simulink model "kiem_chung_dong_hoc"  (R2021a)
settings: Solver=FixedStepAuto  StartTime=0.0  StopTime=5  FixedStep=0.01  RelTol=1e-3
values from neighbouring files (symbols this model uses):
  X = Toado(:,1)    [QuydaoK.m]
  Y = Toado(:,2)    [QuydaoK.m]
  Z = Toado(:,3)    [QuydaoK.m]
undefined symbols (not defined in the file or in its folder): smiData
libraries: sm_lib x36, nesl_utility x13, simulink_extras x12
(part 4 of 4)

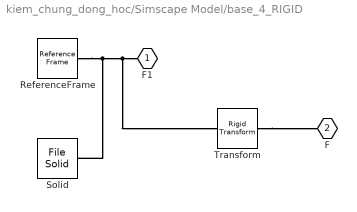
== system kiem_chung_dong_hoc/Simscape Model/base_4_RIGID ==
  ReferenceFrame : sm_lib/Frames and Transforms/Reference Frame
  Solid : sm_lib/Body Elements/File Solid  ExtGeomFileName=base_Default_sldprt.STEP  UnitType=FromFile  ExtGeomFileUnits=m  StepReaderType=HEX  ExportConvexHullGeometry=off  InertiaType=Custom  Mass=smiData.Solid(2).mass  MassUnits=kg  CenterOfMass=smiData.Solid(2).CoM  CenterOfMassUnits=m  MomentsOfInertia=smiData.Solid(2).MoI  MomentsOfInertiaUnits=kg*m^2  ProductsOfInertia=smiData.Solid(2).PoI  ProductsOfInertiaUnits=kg*m^2  BasedOnType=Density  Density=1000  DensityUnits=kg/m^3  DoExposeReferenceFrame=on  SerializedFrames=<Frames/>  GraphicType=FromGeometry  MarkerShape=Sphere  MarkerSize=10  GraphicVisPropType=SimpleVisualProperties  GraphicDiffuseColor=smiData.Solid(2).color  GraphicSpecularColor=[0.5 0.5 0.5 1.0]  GraphicAmbientColor=[0.15 0.15 0.15 1.0]  GraphicEmissiveColor=[0.0 0.0 0.0 1.0]  GraphicShininess=75  GraphicOpacity=smiData.Solid(2).opacity
  Transform : sm_lib/Frames and Transforms/Rigid Transform  TranslationMethod=Cartesian  TranslationStandardOffset=0  TranslationLengthUnit=m  TranslationStandardAxis=+Z  TranslationCartesianOffset=smiData.RigidTransform(3).translation  TranslationROffset=0  TranslationROffsetUnits=m  TranslationZOffset=0  TranslationZOffsetUnits=m  TranslationThetaOffset=0  TranslationThetaOffsetUnits=deg  RotationMethod=ArbitraryAxis  RotationAngleUnits=rad  RotationStandardAxis=+Z  RotationAngle=smiData.RigidTransform(3).angle  RotationArbitraryAxis=smiData.RigidTransform(3).axis  FollAlignAxisA=+X  BaseAlignAxisA=+Y  FollAlignAxisB=+Y  BaseAlignAxisB=+Z  RotationSequenceAxes=FollowerAxes  RotationSequence=XYX  RotationSequenceAngles=[0 0 0]  RotationSequenceAnglesUnits=deg  RotationMatrix=[1 0 0; 0 1 0; 0 0 1]
  F1 : PMIOPort  Side=Left
  F : PMIOPort  Port=2  Side=Right
  connections:
  Solid/RConn1 -- ReferenceFrame/RConn1 -- Transform/LConn1 -- F1/RConn1
  Transform/RConn1 -- F/RConn1

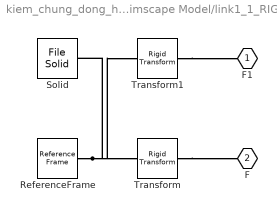
== system kiem_chung_dong_hoc/Simscape Model/link1_1_RIGID ==
  ReferenceFrame : sm_lib/Frames and Transforms/Reference Frame
  Solid : sm_lib/Body Elements/File Solid  ExtGeomFileName=link1_Default_sldprt.STEP  UnitType=FromFile  ExtGeomFileUnits=m  StepReaderType=HEX  ExportConvexHullGeometry=off  InertiaType=Custom  Mass=smiData.Solid(1).mass  MassUnits=kg  CenterOfMass=smiData.Solid(1).CoM  CenterOfMassUnits=m  MomentsOfInertia=smiData.Solid(1).MoI  MomentsOfInertiaUnits=kg*m^2  ProductsOfInertia=smiData.Solid(1).PoI  ProductsOfInertiaUnits=kg*m^2  BasedOnType=Density  Density=1000  DensityUnits=kg/m^3  DoExposeReferenceFrame=on  SerializedFrames=<Frames/>  GraphicType=FromGeometry  MarkerShape=Sphere  MarkerSize=10  GraphicVisPropType=SimpleVisualProperties  GraphicDiffuseColor=smiData.Solid(1).color  GraphicSpecularColor=[0.5 0.5 0.5 1.0]  GraphicAmbientColor=[0.15 0.15 0.15 1.0]  GraphicEmissiveColor=[0.0 0.0 0.0 1.0]  GraphicShininess=75  GraphicOpacity=smiData.Solid(1).opacity
  Transform : sm_lib/Frames and Transforms/Rigid Transform  TranslationMethod=Cartesian  TranslationStandardOffset=0  TranslationLengthUnit=m  TranslationStandardAxis=+Z  TranslationCartesianOffset=smiData.RigidTransform(1).translation  TranslationROffset=0  TranslationROffsetUnits=m  TranslationZOffset=0  TranslationZOffsetUnits=m  TranslationThetaOffset=0  TranslationThetaOffsetUnits=deg  RotationMethod=ArbitraryAxis  RotationAngleUnits=rad  RotationStandardAxis=+Z  RotationAngle=smiData.RigidTransform(1).angle  RotationArbitraryAxis=smiData.RigidTransform(1).axis  FollAlignAxisA=+X  BaseAlignAxisA=+Y  FollAlignAxisB=+Y  BaseAlignAxisB=+Z  RotationSequenceAxes=FollowerAxes  RotationSequence=XYX  RotationSequenceAngles=[0 0 0]  RotationSequenceAnglesUnits=deg  RotationMatrix=[1 0 0; 0 1 0; 0 0 1]
  Transform1 : sm_lib/Frames and Transforms/Rigid Transform  TranslationMethod=Cartesian  TranslationStandardOffset=0  TranslationLengthUnit=m  TranslationStandardAxis=+Z  TranslationCartesianOffset=smiData.RigidTransform(4).translation  TranslationROffset=0  TranslationROffsetUnits=m  TranslationZOffset=0  TranslationZOffsetUnits=m  TranslationThetaOffset=0  TranslationThetaOffsetUnits=deg  RotationMethod=ArbitraryAxis  RotationAngleUnits=rad  RotationStandardAxis=+Z  RotationAngle=smiData.RigidTransform(4).angle  RotationArbitraryAxis=smiData.RigidTransform(4).axis  FollAlignAxisA=+X  BaseAlignAxisA=+Y  FollAlignAxisB=+Y  BaseAlignAxisB=+Z  RotationSequenceAxes=FollowerAxes  RotationSequence=XYX  RotationSequenceAngles=[0 0 0]  RotationSequenceAnglesUnits=deg  RotationMatrix=[1 0 0; 0 1 0; 0 0 1]
  F1 : PMIOPort  Side=Left
  F : PMIOPort  Port=2  Side=Right
  connections:
  Solid/RConn1 -- ReferenceFrame/RConn1 -- Transform/LConn1 -- Transform1/LConn1
  Transform/RConn1 -- F/RConn1
  Transform1/RConn1 -- F1/RConn1

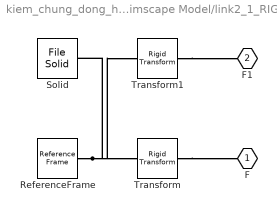
== system kiem_chung_dong_hoc/Simscape Model/link2_1_RIGID ==
  ReferenceFrame : sm_lib/Frames and Transforms/Reference Frame
  Solid : sm_lib/Body Elements/File Solid  ExtGeomFileName=link2_Default_sldprt.STEP  UnitType=FromFile  ExtGeomFileUnits=m  StepReaderType=HEX  ExportConvexHullGeometry=off  InertiaType=Custom  Mass=smiData.Solid(7).mass  MassUnits=kg  CenterOfMass=smiData.Solid(7).CoM  CenterOfMassUnits=m  MomentsOfInertia=smiData.Solid(7).MoI  MomentsOfInertiaUnits=kg*m^2  ProductsOfInertia=smiData.Solid(7).PoI  ProductsOfInertiaUnits=kg*m^2  BasedOnType=Density  Density=1000  DensityUnits=kg/m^3  DoExposeReferenceFrame=on  SerializedFrames=<Frames/>  GraphicType=FromGeometry  MarkerShape=Sphere  MarkerSize=10  GraphicVisPropType=SimpleVisualProperties  GraphicDiffuseColor=smiData.Solid(7).color  GraphicSpecularColor=[0.5 0.5 0.5 1.0]  GraphicAmbientColor=[0.15 0.15 0.15 1.0]  GraphicEmissiveColor=[0.0 0.0 0.0 1.0]  GraphicShininess=75  GraphicOpacity=smiData.Solid(7).opacity
  Transform : sm_lib/Frames and Transforms/Rigid Transform  TranslationMethod=Cartesian  TranslationStandardOffset=0  TranslationLengthUnit=m  TranslationStandardAxis=+Z  TranslationCartesianOffset=smiData.RigidTransform(2).translation  TranslationROffset=0  TranslationROffsetUnits=m  TranslationZOffset=0  TranslationZOffsetUnits=m  TranslationThetaOffset=0  TranslationThetaOffsetUnits=deg  RotationMethod=ArbitraryAxis  RotationAngleUnits=rad  RotationStandardAxis=+Z  RotationAngle=smiData.RigidTransform(2).angle  RotationArbitraryAxis=smiData.RigidTransform(2).axis  FollAlignAxisA=+X  BaseAlignAxisA=+Y  FollAlignAxisB=+Y  BaseAlignAxisB=+Z  RotationSequenceAxes=FollowerAxes  RotationSequence=XYX  RotationSequenceAngles=[0 0 0]  RotationSequenceAnglesUnits=deg  RotationMatrix=[1 0 0; 0 1 0; 0 0 1]
  Transform1 : sm_lib/Frames and Transforms/Rigid Transform  TranslationMethod=Cartesian  TranslationStandardOffset=0  TranslationLengthUnit=m  TranslationStandardAxis=+Z  TranslationCartesianOffset=smiData.RigidTransform(5).translation  TranslationROffset=0  TranslationROffsetUnits=m  TranslationZOffset=0  TranslationZOffsetUnits=m  TranslationThetaOffset=0  TranslationThetaOffsetUnits=deg  RotationMethod=ArbitraryAxis  RotationAngleUnits=rad  RotationStandardAxis=+Z  RotationAngle=smiData.RigidTransform(5).angle  RotationArbitraryAxis=smiData.RigidTransform(5).axis  FollAlignAxisA=+X  BaseAlignAxisA=+Y  FollAlignAxisB=+Y  BaseAlignAxisB=+Z  RotationSequenceAxes=FollowerAxes  RotationSequence=XYX  RotationSequenceAngles=[0 0 0]  RotationSequenceAnglesUnits=deg  RotationMatrix=[1 0 0; 0 1 0; 0 0 1]
  F : PMIOPort  Side=Left
  F1 : PMIOPort  Port=2  Side=Right
  connections:
  Solid/RConn1 -- ReferenceFrame/RConn1 -- Transform/LConn1 -- Transform1/LConn1
  Transform/RConn1 -- F/RConn1
  Transform1/RConn1 -- F1/RConn1

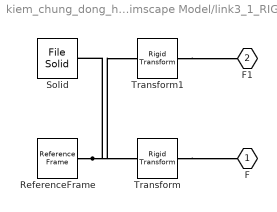
== system kiem_chung_dong_hoc/Simscape Model/link3_1_RIGID ==
  ReferenceFrame : sm_lib/Frames and Transforms/Reference Frame
  Solid : sm_lib/Body Elements/File Solid  ExtGeomFileName=link3_Default_sldprt.STEP  UnitType=FromFile  ExtGeomFileUnits=m  StepReaderType=HEX  ExportConvexHullGeometry=off  InertiaType=Custom  Mass=smiData.Solid(3).mass  MassUnits=kg  CenterOfMass=smiData.Solid(3).CoM  CenterOfMassUnits=m  MomentsOfInertia=smiData.Solid(3).MoI  MomentsOfInertiaUnits=kg*m^2  ProductsOfInertia=smiData.Solid(3).PoI  ProductsOfInertiaUnits=kg*m^2  BasedOnType=Density  Density=1000  DensityUnits=kg/m^3  DoExposeReferenceFrame=on  SerializedFrames=<Frames/>  GraphicType=FromGeometry  MarkerShape=Sphere  MarkerSize=10  GraphicVisPropType=SimpleVisualProperties  GraphicDiffuseColor=smiData.Solid(3).color  GraphicSpecularColor=[0.5 0.5 0.5 1.0]  GraphicAmbientColor=[0.15 0.15 0.15 1.0]  GraphicEmissiveColor=[0.0 0.0 0.0 1.0]  GraphicShininess=75  GraphicOpacity=smiData.Solid(3).opacity
  Transform : sm_lib/Frames and Transforms/Rigid Transform  TranslationMethod=Cartesian  TranslationStandardOffset=0  TranslationLengthUnit=m  TranslationStandardAxis=+Z  TranslationCartesianOffset=smiData.RigidTransform(6).translation  TranslationROffset=0  TranslationROffsetUnits=m  TranslationZOffset=0  TranslationZOffsetUnits=m  TranslationThetaOffset=0  TranslationThetaOffsetUnits=deg  RotationMethod=ArbitraryAxis  RotationAngleUnits=rad  RotationStandardAxis=+Z  RotationAngle=smiData.RigidTransform(6).angle  RotationArbitraryAxis=smiData.RigidTransform(6).axis  FollAlignAxisA=+X  BaseAlignAxisA=+Y  FollAlignAxisB=+Y  BaseAlignAxisB=+Z  RotationSequenceAxes=FollowerAxes  RotationSequence=XYX  RotationSequenceAngles=[0 0 0]  RotationSequenceAnglesUnits=deg  RotationMatrix=[1 0 0; 0 1 0; 0 0 1]
  Transform1 : sm_lib/Frames and Transforms/Rigid Transform  TranslationMethod=Cartesian  TranslationStandardOffset=0  TranslationLengthUnit=m  TranslationStandardAxis=+Z  TranslationCartesianOffset=smiData.RigidTransform(7).translation  TranslationROffset=0  TranslationROffsetUnits=m  TranslationZOffset=0  TranslationZOffsetUnits=m  TranslationThetaOffset=0  TranslationThetaOffsetUnits=deg  RotationMethod=ArbitraryAxis  RotationAngleUnits=rad  RotationStandardAxis=+Z  RotationAngle=smiData.RigidTransform(7).angle  RotationArbitraryAxis=smiData.RigidTransform(7).axis  FollAlignAxisA=+X  BaseAlignAxisA=+Y  FollAlignAxisB=+Y  BaseAlignAxisB=+Z  RotationSequenceAxes=FollowerAxes  RotationSequence=XYX  RotationSequenceAngles=[0 0 0]  RotationSequenceAnglesUnits=deg  RotationMatrix=[1 0 0; 0 1 0; 0 0 1]
  F : PMIOPort  Side=Left
  F1 : PMIOPort  Port=2  Side=Right
  connections:
  Solid/RConn1 -- ReferenceFrame/RConn1 -- Transform/LConn1 -- Transform1/LConn1
  Transform/RConn1 -- F/RConn1
  Transform1/RConn1 -- F1/RConn1

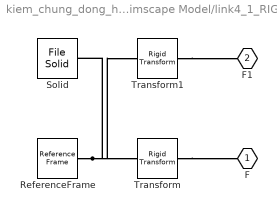
== system kiem_chung_dong_hoc/Simscape Model/link4_1_RIGID ==
  ReferenceFrame : sm_lib/Frames and Transforms/Reference Frame
  Solid : sm_lib/Body Elements/File Solid  ExtGeomFileName=link4_Default_sldprt.STEP  UnitType=FromFile  ExtGeomFileUnits=m  StepReaderType=HEX  ExportConvexHullGeometry=off  InertiaType=Custom  Mass=smiData.Solid(4).mass  MassUnits=kg  CenterOfMass=smiData.Solid(4).CoM  CenterOfMassUnits=m  MomentsOfInertia=smiData.Solid(4).MoI  MomentsOfInertiaUnits=kg*m^2  ProductsOfInertia=smiData.Solid(4).PoI  ProductsOfInertiaUnits=kg*m^2  BasedOnType=Density  Density=1000  DensityUnits=kg/m^3  DoExposeReferenceFrame=on  SerializedFrames=<Frames/>  GraphicType=FromGeometry  MarkerShape=Sphere  MarkerSize=10  GraphicVisPropType=SimpleVisualProperties  GraphicDiffuseColor=smiData.Solid(4).color  GraphicSpecularColor=[0.5 0.5 0.5 1.0]  GraphicAmbientColor=[0.15 0.15 0.15 1.0]  GraphicEmissiveColor=[0.0 0.0 0.0 1.0]  GraphicShininess=75  GraphicOpacity=smiData.Solid(4).opacity
  Transform : sm_lib/Frames and Transforms/Rigid Transform  TranslationMethod=Cartesian  TranslationStandardOffset=0  TranslationLengthUnit=m  TranslationStandardAxis=+Z  TranslationCartesianOffset=smiData.RigidTransform(8).translation  TranslationROffset=0  TranslationROffsetUnits=m  TranslationZOffset=0  TranslationZOffsetUnits=m  TranslationThetaOffset=0  TranslationThetaOffsetUnits=deg  RotationMethod=ArbitraryAxis  RotationAngleUnits=rad  RotationStandardAxis=+Z  RotationAngle=smiData.RigidTransform(8).angle  RotationArbitraryAxis=smiData.RigidTransform(8).axis  FollAlignAxisA=+X  BaseAlignAxisA=+Y  FollAlignAxisB=+Y  BaseAlignAxisB=+Z  RotationSequenceAxes=FollowerAxes  RotationSequence=XYX  RotationSequenceAngles=[0 0 0]  RotationSequenceAnglesUnits=deg  RotationMatrix=[1 0 0; 0 1 0; 0 0 1]
  Transform1 : sm_lib/Frames and Transforms/Rigid Transform  TranslationMethod=Cartesian  TranslationStandardOffset=0  TranslationLengthUnit=m  TranslationStandardAxis=+Z  TranslationCartesianOffset=smiData.RigidTransform(9).translation  TranslationROffset=0  TranslationROffsetUnits=m  TranslationZOffset=0  TranslationZOffsetUnits=m  TranslationThetaOffset=0  TranslationThetaOffsetUnits=deg  RotationMethod=ArbitraryAxis  RotationAngleUnits=rad  RotationStandardAxis=+Z  RotationAngle=smiData.RigidTransform(9).angle  RotationArbitraryAxis=smiData.RigidTransform(9).axis  FollAlignAxisA=+X  BaseAlignAxisA=+Y  FollAlignAxisB=+Y  BaseAlignAxisB=+Z  RotationSequenceAxes=FollowerAxes  RotationSequence=XYX  RotationSequenceAngles=[0 0 0]  RotationSequenceAnglesUnits=deg  RotationMatrix=[1 0 0; 0 1 0; 0 0 1]
  F : PMIOPort  Side=Left
  F1 : PMIOPort  Port=2  Side=Right
  connections:
  Solid/RConn1 -- ReferenceFrame/RConn1 -- Transform/LConn1 -- Transform1/LConn1
  Transform/RConn1 -- F/RConn1
  Transform1/RConn1 -- F1/RConn1

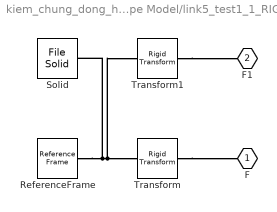
== system kiem_chung_dong_hoc/Simscape Model/link5_test1_1_RIGID ==
  ReferenceFrame : sm_lib/Frames and Transforms/Reference Frame
  Solid : sm_lib/Body Elements/File Solid  ExtGeomFileName=link5_test1_Default_sldprt.STEP  UnitType=FromFile  ExtGeomFileUnits=m  StepReaderType=HEX  ExportConvexHullGeometry=off  InertiaType=Custom  Mass=smiData.Solid(5).mass  MassUnits=kg  CenterOfMass=smiData.Solid(5).CoM  CenterOfMassUnits=m  MomentsOfInertia=smiData.Solid(5).MoI  MomentsOfInertiaUnits=kg*m^2  ProductsOfInertia=smiData.Solid(5).PoI  ProductsOfInertiaUnits=kg*m^2  BasedOnType=Density  Density=1000  DensityUnits=kg/m^3  DoExposeReferenceFrame=on  SerializedFrames=<Frames/>  GraphicType=FromGeometry  MarkerShape=Sphere  MarkerSize=10  GraphicVisPropType=SimpleVisualProperties  GraphicDiffuseColor=smiData.Solid(5).color  GraphicSpecularColor=[0.5 0.5 0.5 1.0]  GraphicAmbientColor=[0.15 0.15 0.15 1.0]  GraphicEmissiveColor=[0.0 0.0 0.0 1.0]  GraphicShininess=75  GraphicOpacity=smiData.Solid(5).opacity
  Transform : sm_lib/Frames and Transforms/Rigid Transform  TranslationMethod=Cartesian  TranslationStandardOffset=0  TranslationLengthUnit=m  TranslationStandardAxis=+Z  TranslationCartesianOffset=smiData.RigidTransform(10).translation  TranslationROffset=0  TranslationROffsetUnits=m  TranslationZOffset=0  TranslationZOffsetUnits=m  TranslationThetaOffset=0  TranslationThetaOffsetUnits=deg  RotationMethod=ArbitraryAxis  RotationAngleUnits=rad  RotationStandardAxis=+Z  RotationAngle=smiData.RigidTransform(10).angle  RotationArbitraryAxis=smiData.RigidTransform(10).axis  FollAlignAxisA=+X  BaseAlignAxisA=+Y  FollAlignAxisB=+Y  BaseAlignAxisB=+Z  RotationSequenceAxes=FollowerAxes  RotationSequence=XYX  RotationSequenceAngles=[0 0 0]  RotationSequenceAnglesUnits=deg  RotationMatrix=[1 0 0; 0 1 0; 0 0 1]
  Transform1 : sm_lib/Frames and Transforms/Rigid Transform  TranslationMethod=Cartesian  TranslationStandardOffset=0  TranslationLengthUnit=m  TranslationStandardAxis=+Z  TranslationCartesianOffset=smiData.RigidTransform(11).translation  TranslationROffset=0  TranslationROffsetUnits=m  TranslationZOffset=0  TranslationZOffsetUnits=m  TranslationThetaOffset=0  TranslationThetaOffsetUnits=deg  RotationMethod=ArbitraryAxis  RotationAngleUnits=rad  RotationStandardAxis=+Z  RotationAngle=smiData.RigidTransform(11).angle  RotationArbitraryAxis=smiData.RigidTransform(11).axis  FollAlignAxisA=+X  BaseAlignAxisA=+Y  FollAlignAxisB=+Y  BaseAlignAxisB=+Z  RotationSequenceAxes=FollowerAxes  RotationSequence=XYX  RotationSequenceAngles=[0 0 0]  RotationSequenceAnglesUnits=deg  RotationMatrix=[1 0 0; 0 1 0; 0 0 1]
  F : PMIOPort  Side=Left
  F1 : PMIOPort  Port=2  Side=Right
  connections:
  Solid/RConn1 -- ReferenceFrame/RConn1 -- Transform/LConn1 -- Transform1/LConn1
  Transform/RConn1 -- F/RConn1
  Transform1/RConn1 -- F1/RConn1

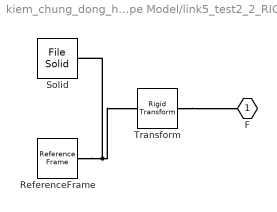
== system kiem_chung_dong_hoc/Simscape Model/link5_test2_2_RIGID ==
  ReferenceFrame : sm_lib/Frames and Transforms/Reference Frame
  Solid : sm_lib/Body Elements/File Solid  ExtGeomFileName=link5_test2_Default_sldprt.STEP  UnitType=FromFile  ExtGeomFileUnits=m  StepReaderType=HEX  ExportConvexHullGeometry=off  InertiaType=Custom  Mass=smiData.Solid(6).mass  MassUnits=kg  CenterOfMass=smiData.Solid(6).CoM  CenterOfMassUnits=m  MomentsOfInertia=smiData.Solid(6).MoI  MomentsOfInertiaUnits=kg*m^2  ProductsOfInertia=smiData.Solid(6).PoI  ProductsOfInertiaUnits=kg*m^2  BasedOnType=Density  Density=1000  DensityUnits=kg/m^3  DoExposeReferenceFrame=on  SerializedFrames=<Frames/>  GraphicType=FromGeometry  MarkerShape=Sphere  MarkerSize=10  GraphicVisPropType=SimpleVisualProperties  GraphicDiffuseColor=smiData.Solid(6).color  GraphicSpecularColor=[0.5 0.5 0.5 1.0]  GraphicAmbientColor=[0.15 0.15 0.15 1.0]  GraphicEmissiveColor=[0.0 0.0 0.0 1.0]  GraphicShininess=75  GraphicOpacity=smiData.Solid(6).opacity
  Transform : sm_lib/Frames and Transforms/Rigid Transform  TranslationMethod=Cartesian  TranslationStandardOffset=0  TranslationLengthUnit=m  TranslationStandardAxis=+Z  TranslationCartesianOffset=smiData.RigidTransform(12).translation  TranslationROffset=0  TranslationROffsetUnits=m  TranslationZOffset=0  TranslationZOffsetUnits=m  TranslationThetaOffset=0  TranslationThetaOffsetUnits=deg  RotationMethod=ArbitraryAxis  RotationAngleUnits=rad  RotationStandardAxis=+Z  RotationAngle=smiData.RigidTransform(12).angle  RotationArbitraryAxis=smiData.RigidTransform(12).axis  FollAlignAxisA=+X  BaseAlignAxisA=+Y  FollAlignAxisB=+Y  BaseAlignAxisB=+Z  RotationSequenceAxes=FollowerAxes  RotationSequence=XYX  RotationSequenceAngles=[0 0 0]  RotationSequenceAnglesUnits=deg  RotationMatrix=[1 0 0; 0 1 0; 0 0 1]
  F : PMIOPort  Side=Left
  connections:
  Solid/RConn1 -- ReferenceFrame/RConn1 -- Transform/LConn1
  Transform/RConn1 -- F/RConn1

== matlab function kiem_chung_dong_hoc/Dong hoc nghich/DONG HOC NGHICH ==
  data: P_EE input; the1 output; the2 output; yaw input; pitch input; roll input; the3 output; the4 output; the5 output; the6 output
% Programmed by Nguyen Ngoc Thien
% Date: 14/07/2022
function [the1,the2,the3,the4,the5,the6] = IK_6DOF(P_EE,yaw,pitch,roll)
%% Thong so cua Robot 6DoF
L2=270; L3=295; L4=80; d1=75; d2=335; d3=90;
% A = [0 0 0 0 0 0;0 0 0 0 0 0;0 0 0 0 0 0;0 0 0 0 0 0;0 0 0 0 0 0;0 0 0 0 0 0;0 0 0 0 0 0;0 0 0 0 0 0];
%% Bo nghiem cua loi giai dong hoc nghich
i = 2;
%% Huong cua Robot
r11 = cosd(yaw)*cosd(pitch);
r12 = cosd(yaw)*sind(pitch)*sind(roll) - sind(yaw)*cosd(roll);
r13 = cosd(yaw)*sind(pitch)*cosd(roll) + sind(yaw)*sind(roll);
r21 = sind(yaw)*cosd(pitch);
r22 = sind(yaw)*sind(pitch)*sind(roll) + cosd(yaw)*cosd(roll);
r23 = sind(yaw)*sind(pitch)*cosd(roll) - cosd(yaw)*sind(roll);
r31 = -sind(pitch);
r32 = cosd(pitch)*sind(roll);
r33 = cosd(pitch)*cosd(roll);
Px = P_EE(1) - L4*r13;
Py = P_EE(2) - L4*r23;
Pz = P_EE(3) - L4*r33;
%% Tinh theta1
s1 = Py/(sqrt(Px^2+Py^2));
c1 = sqrt(1-s1^2);
t1 = [atan2d(s1,c1);
      atan2d(s1,-c1);];
if (i >= 1 && i <= 4)
    the1 = t1(1);
end
if (i >= 5 && i <= 8)
    the1 = t1(2);
end
% for i1 = 1:8
%     A(i1,1) = the1;
% end
%% Tinh theta3
K = ((Px*cosd(the1)+Py*sind(the1)-d1)^2+(Pz-d2)^2-d3^2-L2^2-L3^2)/(2*L2);
t3=[atan2d(d3,L3) - atan2d(K,sqrt(d3^2+L3^2-K^2));
    atan2d(d3,L3) - atan2d(K,-sqrt(d3^2+L3^2-K^2));];
if (i==1 || i==2 || i==5 || i==6)
    the3 = t3(1);
end
if (i==3 || i==4 || i==7 || i==8)
    the3 = t3(2);
end
% for i3 = 1:8
%     A(i3,3) = the3;
% end
%% Tinh theta2
a3=Px*cosd(the1)+Py*sind(the1)-d1;
b3=Pz-d2;
a11=L3*cosd(the3) + d3*sind(the3);
a12=L2 + d3*cosd(the3) - L3*sind(the3);
a21=d3*cosd(the3) - L3*sind(the3) + L2;
a22=-d3*sind(the3) - L3*cosd(the3);
c2=(a3*a22-b3*a12)/(a11*a22-a21*a12);
s2=(a11*b3-a21*a3)/(a11*a22-a21*a12);
the2 = atan2d(s2,c2);
% for i2 = 1:8
%     A(i2,2) = the2;
% end
%% Tinh theta5
c5= r13*cosd(the2 + the3)*cosd(the1) - r33*sind(the2 + the3) + r23*cosd(the2 + the3)*sind(the1);
s5= sqrt(1-c5^2);
t5=[atan2d(s5,c5);
    atan2d(-s5,c5);];
if (i==1 || i==3 || i==5 || i==7)
    the5 = t5(1);
end
if (i==2 || i==4 || i==6 || i==8)
    the5 = t5(2);
end
% for i5 = 1:8
%     A(i5,5) = the5;
% end
%% Tinh theta4
s4=(r23*cosd(the1) - r13*sind(the1))/sind(the5);
c4=-(r33*cosd(the2 + the3) + r13*sind(the2 + the3)*cosd(the1) + r23*sind(the2 + the3)*sind(the1))/sind(the5);
the4 = atan2d(s4,c4);
% for i4 = 1:8
%     A(i4,4) = the4;
% end
%% Tinh theta6
s6= -(r12*cosd(the2 + the3)*cosd(the1) - r32*sind(the2 + the3) + r22*cosd(the2 + the3)*sind(the1))/sind(the5);
c6=(r11*cosd(the2 + the3)*cosd(the1) - r31*sind(the2 + the3) + r21*cosd(the2 + the3)*sind(the1))/sind(the5);
the6 = atan2d(s6,c6);
% for i6 = 1:8
%     A(i6,6) = the6;
% end
end

== matlab function kiem_chung_dong_hoc/Dong hoc thuan/DONG HOC THUAN ==
  data: the1 input; P_EE output; the2 input; the3 input; the4 input; the5 input; the6 input; yaw output; pitch output; roll output
% Programmed by: Nguyen Ngoc Thien
% Date: 14/07/2022
function [P_EE,yaw,pitch,roll]=FK_6DOF(the1,the2,the3,the4,the5,the6)
%% Thong so cua Robot 6DoF
L2=270; L3=295; L4=80; d1=75; d2=335; d3=90;
%% Loi giai dong hoc thuan
P_EE = [cosd(the1)*(d1 + L3*cosd(the2 + the3) + d3*sind(the2 + the3) + L2*sind(the2)) + L4*(cosd(the1)*(cosd(the2 + the3)*cosd(the5) - sind(the2 + the3)*cosd(the4)*sind(the5)) - sind(the1)*sind(the4)*sind(the5));
        sind(the1)*(d1 + L3*cosd(the2 + the3) + d3*sind(the2 + the3) + L2*sind(the2)) + L4*(sind(the1)*(cosd(the2 + the3)*cosd(the5) - sind(the2 + the3)*cosd(the4)*sind(the5)) + cosd(the1)*sind(the4)*sind(the5));
        d2 - L3*sind(the2 + the3) + d3*cosd(the2 + the3) + L2*cosd(the2) - L4*(sind(the2 + the3)*cosd(the5) + cosd(the2 + the3)*cosd(the4)*sind(the5));
        1;];
%% Thanh phan huong cua Robot 6DoF
r11= sind(the6)*(cosd(the4)*sind(the1) - sind(the4)*(cosd(the1)*cosd(the2)*sind(the3) + cosd(the1)*cosd(the3)*sind(the2))) + cosd(the6)*(cosd(the5)*(sind(the1)*sind(the4) + cosd(the4)*(cosd(the1)*cosd(the2)*sind(the3) + cosd(the1)*cosd(the3)*sind(the2))) - sind(the5)*(cosd(the1)*sind(the2)*sind(the3) - cosd(the1)*cosd(the2)*cosd(the3)));
r12= cosd(the6)*(cosd(the4)*sind(the1) - sind(the4)*(cosd(the1)*cosd(the2)*sind(the3) + cosd(the1)*cosd(the3)*sind(the2))) - sind(the6)*(cosd(the5)*(sind(the1)*sind(the4) + cosd(the4)*(cosd(the1)*cosd(the2)*sind(the3) + cosd(the1)*cosd(the3)*sind(the2))) - sind(the5)*(cosd(the1)*sind(the2)*sind(the3) - cosd(the1)*cosd(the2)*cosd(the3)));
r13= - sind(the5)*(sind(the1)*sind(the4) + cosd(the4)*(cosd(the1)*cosd(the2)*sind(the3) + cosd(the1)*cosd(the3)*sind(the2))) - cosd(the5)*(cosd(the1)*sind(the2)*sind(the3) - cosd(the1)*cosd(the2)*cosd(the3));
r21= - sind(the6)*(cosd(the1)*cosd(the4) + sind(the4)*(cosd(the2)*sind(the1)*sind(the3) + cosd(the3)*sind(the1)*sind(the2))) - cosd(the6)*(cosd(the5)*(cosd(the1)*sind(the4) - cosd(the4)*(cosd(the2)*sind(the1)*sind(the3) + cosd(the3)*sind(the1)*sind(the2))) + sind(the5)*(sind(the1)*sind(the2)*sind(the3) - cosd(the2)*cosd(the3)*sind(the1)));
r22= sind(the6)*(cosd(the5)*(cosd(the1)*sind(the4) - cosd(the4)*(cosd(the2)*sind(the1)*sind(the3) + cosd(the3)*sind(the1)*sind(the2))) + sind(the5)*(sind(the1)*sind(the2)*sind(the3) - cosd(the2)*cosd(the3)*sind(the1))) - cosd(the6)*(cosd(the1)*cosd(the4) + sind(the4)*(cosd(the2)*sind(the1)*sind(the3) + cosd(the3)*sind(the1)*sind(the2)));
r23= sind(the5)*(cosd(the1)*sind(the4) - cosd(the4)*(cosd(the2)*sind(the1)*sind(the3) + cosd(the3)*sind(the1)*sind(the2))) - cosd(the5)*(sind(the1)*sind(the2)*sind(the3) - cosd(the2)*cosd(the3)*sind(the1));
r31= - cosd(the6)*(sind(the2 + the3)*sind(the5) - cosd(the2 + the3)*cosd(the4)*cosd(the5)) - cosd(the2 + the3)*sind(the4)*sind(the6);
r32= sind(the6)*(sind(the2 + the3)*sind(the5) - cosd(the2 + the3)*cosd(the4)*cosd(the5)) - cosd(the2 + the3)*cosd(the6)*sind(the4);
r33= - sind(the2 + the3)*cosd(the5) - cosd(the2 + the3)*cosd(the4)*sind(the5);
%% Cac goc quay Euler Yaw Pitch Roll
pitch = atan2d(-r31,sqrt(r11^2+r21^2));
yaw = atan2d(r21/cosd(pitch),r11/cosd(pitch));
roll = atan2d(r32/cosd(pitch),r33/cosd(pitch));
end

== matlab function kiem_chung_dong_hoc/Dong hoc nghich1/DONG HOC NGHICH ==
  data: P_EE input; the1 output; the2 output; yaw input; pitch input; roll input; the3 output; the4 output; the5 output; the6 output
% Programmed by Nguyen Ngoc Thien
% Date: 14/07/2022
function [the1,the2,the3,the4,the5,the6] = IK_6DOF(P_EE,yaw,pitch,roll)
%% Thong so cua Robot 6DoF
L2=270; L3=295; L4=80; d1=75; d2=335; d3=90;
% A = [0 0 0 0 0 0;0 0 0 0 0 0;0 0 0 0 0 0;0 0 0 0 0 0;0 0 0 0 0 0;0 0 0 0 0 0;0 0 0 0 0 0;0 0 0 0 0 0];
%% Bo nghiem cua loi giai dong hoc nghich
i = 2;
%% Huong cua Robot
r11 = cosd(yaw)*cosd(pitch);
r12 = cosd(yaw)*sind(pitch)*sind(roll) - sind(yaw)*cosd(roll);
r13 = cosd(yaw)*sind(pitch)*cosd(roll) + sind(yaw)*sind(roll);
r21 = sind(yaw)*cosd(pitch);
r22 = sind(yaw)*sind(pitch)*sind(roll) + cosd(yaw)*cosd(roll);
r23 = sind(yaw)*sind(pitch)*cosd(roll) - cosd(yaw)*sind(roll);
r31 = -sind(pitch);
r32 = cosd(pitch)*sind(roll);
r33 = cosd(pitch)*cosd(roll);
Px = P_EE(1) - L4*r13;
Py = P_EE(2) - L4*r23;
Pz = P_EE(3) - L4*r33;
%% Tinh theta1
s1 = Py/(sqrt(Px^2+Py^2));
c1 = sqrt(1-s1^2);
t1 = [atan2d(s1,c1);
      atan2d(s1,-c1);];
if (i >= 1 && i <= 4)
    the1 = t1(1);
end
if (i >= 5 && i <= 8)
    the1 = t1(2);
end
% for i1 = 1:8
%     A(i1,1) = the1;
% end
%% Tinh theta3
K = ((Px*cosd(the1)+Py*sind(the1)-d1)^2+(Pz-d2)^2-d3^2-L2^2-L3^2)/(2*L2);
t3=[atan2d(d3,L3) - atan2d(K,sqrt(d3^2+L3^2-K^2));
    atan2d(d3,L3) - atan2d(K,-sqrt(d3^2+L3^2-K^2));];
if (i==1 || i==2 || i==5 || i==6)
    the3 = t3(1);
end
if (i==3 || i==4 || i==7 || i==8)
    the3 = t3(2);
end
% for i3 = 1:8
%     A(i3,3) = the3;
% end
%% Tinh theta2
a3=Px*cosd(the1)+Py*sind(the1)-d1;
b3=Pz-d2;
a11=L3*cosd(the3) + d3*sind(the3);
a12=L2 + d3*cosd(the3) - L3*sind(the3);
a21=d3*cosd(the3) - L3*sind(the3) + L2;
a22=-d3*sind(the3) - L3*cosd(the3);
c2=(a3*a22-b3*a12)/(a11*a22-a21*a12);
s2=(a11*b3-a21*a3)/(a11*a22-a21*a12);
the2 = atan2d(s2,c2);
% for i2 = 1:8
%     A(i2,2) = the2;
% end
%% Tinh theta5
c5= r13*cosd(the2 + the3)*cosd(the1) - r33*sind(the2 + the3) + r23*cosd(the2 + the3)*sind(the1);
s5= sqrt(1-c5^2);
t5=[atan2d(s5,c5);
    atan2d(-s5,c5);];
if (i==1 || i==3 || i==5 || i==7)
    the5 = t5(1);
end
if (i==2 || i==4 || i==6 || i==8)
    the5 = t5(2);
end
% for i5 = 1:8
%     A(i5,5) = the5;
% end
%% Tinh theta4
s4=(r23*cosd(the1) - r13*sind(the1))/sind(the5);
c4=-(r33*cosd(the2 + the3) + r13*sind(the2 + the3)*cosd(the1) + r23*sind(the2 + the3)*sind(the1))/sind(the5);
the4 = atan2d(s4,c4);
% for i4 = 1:8
%     A(i4,4) = the4;
% end
%% Tinh theta6
s6= -(r12*cosd(the2 + the3)*cosd(the1) - r32*sind(the2 + the3) + r22*cosd(the2 + the3)*sind(the1))/sind(the5);
c6=(r11*cosd(the2 + the3)*cosd(the1) - r31*sind(the2 + the3) + r21*cosd(the2 + the3)*sind(the1))/sind(the5);
the6 = atan2d(s6,c6);
% for i6 = 1:8
%     A(i6,6) = the6;
% end
end
